simulink model "demo_interconnect_new"  (Simulink 7.4)
settings: Solver=ode45  StartTime=0.0  StopTime=100  RelTol=1e-3
undefined symbols (not defined in the file): ROACH
libraries: xbsIndex_r4 x58, isi_correlator_lib x22, xps_library x13, casper_library x8, dspsigops x8
settings Model: Creator=wjm  LastModifiedBy=wjm
settings OptimizationCC: InitFltsAndDblsToZero=on

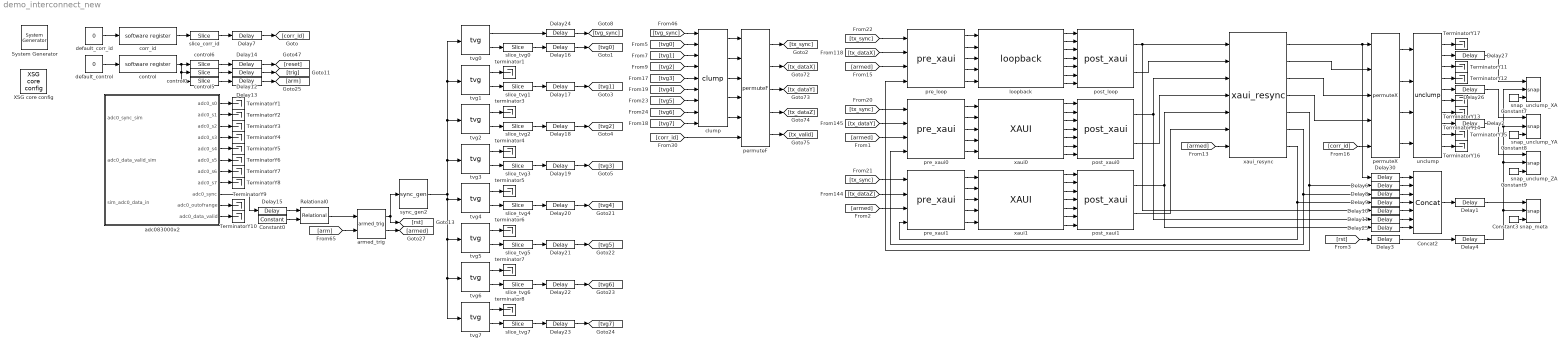
== system demo_interconnect_new ==
  " System Generator" : xbsIndex_r4/ System Generator  Tag=genX  SystemSampleTime=-1  xilinxfamily=virtex5  part=xc5vsx95t  speed=-1  package=ff1136  synthesis_tool=XST  clock_wrapper=Clock Enables  directory=./demo_interconnect_new/sysgen  testbench=off  simulink_period=1  sysclk_period=5  dcm_input_clock_period=100  incr_netlist=off  trim_vbits=Everywhere in SubSystem  dbl_ovrd=According to Block Masks  core_generation=According to Block Masks  run_coregen=off  deprecated_control=off  eval_field=0  block_type=sysgen
      settings: block_version=10.1.1
  Concat2 : xbsIndex_r4/Concat  num_inputs=7  dbl_ovrd=off  block_type=concat
      settings: block_version=11.3
  Constant0 : xbsIndex_r4/Constant  arith_type=Unsigned  const=0  n_bits=4  bin_pt=0  explicit_period=on  period=1  equ=P=C  opselect=C  inp2=PCIN>>17  opr=+  inp1=P  carry=CIN  dbl_ovrd=off  block_type=constant
  Constant{3,7..9} (4 alike) : xbsIndex_r4/Constant  arith_type=Boolean  const=1  n_bits=1  bin_pt=0  explicit_period=on  period=1  equ=P=C  opselect=C  inp2=PCIN>>17  opr=+  inp1=P  carry=CIN  dbl_ovrd=off  block_type=constant
      settings: block_version=10.1.1
  Delay{1..2,4,12..24,26..27} (18 alike) : xbsIndex_r4/Delay  en=off  latency=1  dbl_ovrd=off  reg_retiming=on  block_type=delay
  Delay{3,6,8..11,25,30} (8 alike) : xbsIndex_r4/Delay  en=off  latency=3  dbl_ovrd=off  reg_retiming=on  block_type=delay
  Delay7 : xbsIndex_r4/Delay  en=off  latency=0  dbl_ovrd=off  reg_retiming=on  block_type=delay
  Relational0 : xbsIndex_r4/Relational  mode=a!=b  en=off  latency=1  dbl_ovrd=off  block_type=relational
      settings: xl_area=[0, 0, 0, 0, 0, 0, 0]  block_version=10.1.3
  TerminatorY{1..17} (17 alike) : Terminator
  XSG core config : xps_library/XSG core config  Tag=xps:xsg  SystemSampleTime=-1  hw_sys=ROACH:sx95t  ibob_linux=off  clk_src=adc0_clk  iBOB_clk_src=sys_clk  BEE2_ctrl_clk_src=sys_clk  BEE2_usr_clk_src=sys_clk  ROACH_clk_src=adc0_clk  CORR_clk_src=sys_clk  gpio_clk_io_group=iBOB:sma  gpio_clk_bit_index=0  clk_rate=200  sample_period=1  synthesis_tool=XST  mpc_type=powerpc440_ext
  adc083000x2 : Subsystem  Tag=xps:adc083000x2  AncestorBlock=xps_library/adc083000x2  mask(adc_083000x2){use_adc0=on, use_adc1=off, demux_adc=off, clock_sync=off, verbose=off, using_ctrl=off, adc_clk_rate=800, sample_period=1, bit_width=8}
      mask prompts: use_adc0 "Use ZD0K0?"; use_adc1 "Use ZDOK1?"; demux_adc "Demux ADCs by 2?"; clock_sync "Interleave 2 ADC boards?"; verbose "Verbose Block Creation?"; using_ctrl "Add ports for control registers?"; adc_clk_rate "ADC clock rate (MHz)"; sample_period "Sample Period"; bit_width "Output Bit Width"
      mask help:
      | The ADC block converts analog inputs to digital outputs.
      | Every clock cycle, the inputs are sampled and digitized to
      | 8 bit binary point numbers in the range of [-1, 1).
      |
      | Online block-specific documentation: http://casper.berkeley.edu/wiki/Adc083000
      mask init:
      | adc083000_mask;
      mask Help: eval('xlWeb([getenv(''MLIB_ROOT''), ''\doc\html\sys_adc\sys_adc.html''])')
  armed_trig : isi_correlator_lib/armed_trig  SystemSampleTime=-1
  clump : isi_correlator_lib/clump  SystemSampleTime=-1
  control : xps_library/software register  Tag=xps:sw_reg  SystemSampleTime=-1  io_dir=From Processor  arith_type=Unsigned  bitwidth=32  bin_pt=0  sample_period=1  gw_name=demo_interconnect_new_control_user_data_out
  control0 : xbsIndex_r4/Slice  nbits=1  boolean_output=on  mode=Lower Bit Location + Width  bit1=0  base1=MSB of Input  bit0=0  base0=LSB of Input  dbl_ovrd=off  block_type=slice
      settings: infoedit="Extracts a given range of bits from each input sample and presents it at the output.  The output type is ordinarily unsigned with binary point at zero, but can be Boolean when the slice is one bit wide.<P><P>Hardware notes: In hardware this block costs nothing."  block_version=10.1.3
  control5 : xbsIndex_r4/Slice  nbits=1  boolean_output=on  mode=Lower Bit Location + Width  bit1=0  base1=MSB of Input  bit0=1  base0=LSB of Input  dbl_ovrd=off  block_type=slice
      settings: infoedit="Extracts a given range of bits from each input sample and presents it at the output.  The output type is ordinarily unsigned with binary point at zero, but can be Boolean when the slice is one bit wide.<P><P>Hardware notes: In hardware this block costs nothing."  block_version=10.1.3
  control6 : xbsIndex_r4/Slice  nbits=1  boolean_output=on  mode=Lower Bit Location + Width  bit1=0  base1=MSB of Input  bit0=2  base0=LSB of Input  dbl_ovrd=off  block_type=slice
      settings: infoedit="Extracts a given range of bits from each input sample and presents it at the output.  The output type is ordinarily unsigned with binary point at zero, but can be Boolean when the slice is one bit wide.<P><P>Hardware notes: In hardware this block costs nothing."  block_version=10.1.3
  corr_id : xps_library/software register  Tag=xps:sw_reg  SystemSampleTime=-1  io_dir=From Processor  arith_type=Unsigned  bitwidth=32  bin_pt=0  sample_period=1  gw_name=demo_interconnect_new_corr_id_user_data_out
  default_control : Constant  Value=0  OutDataType=sfix(16)  OutScaling=2^0  SampleTime=1
  default_corr_id : Constant  Value=0  OutDataType=sfix(16)  OutScaling=2^0  SampleTime=1
  loopback : isi_correlator_lib/loopback  SystemSampleTime=-1
  permuteF : isi_correlator_lib/permuteF  SystemSampleTime=-1  latency=3
  permuteX : isi_correlator_lib/permuteX  SystemSampleTime=-1  latency=3
  post_loop : isi_correlator_lib/post_xaui  SystemSampleTime=-1
  post_xaui0 : isi_correlator_lib/post_xaui  SystemSampleTime=-1
  post_xaui1 : isi_correlator_lib/post_xaui  SystemSampleTime=-1
  pre_loop : isi_correlator_lib/pre_xaui  SystemSampleTime=-1
  pre_xaui0 : isi_correlator_lib/pre_xaui  SystemSampleTime=-1
  pre_xaui1 : isi_correlator_lib/pre_xaui  SystemSampleTime=-1
  slice_corr_id : xbsIndex_r4/Slice  nbits=2  boolean_output=off  mode=Lower Bit Location + Width  bit1=0  base1=MSB of Input  bit0=0  base0=LSB of Input  dbl_ovrd=off  block_type=slice
      settings: infoedit="Extracts a given range of bits from each input sample and presents it at the output.  The output type is ordinarily unsigned with binary point at zero, but can be Boolean when the slice is one bit wide.<P><P>Hardware notes: In hardware this block costs nothing."  block_version=10.1.3
  slice_tvg{0..7} (8 alike) : xbsIndex_r4/Slice  nbits=8  boolean_output=off  mode=Lower Bit Location + Width  bit1=0  base1=MSB of Input  bit0=0  base0=LSB of Input  dbl_ovrd=off  block_type=slice
      settings: block_version=10.1.3
  snap_meta : casper_library/Scopes/snap  SystemSampleTime=-1  nsamples=13
  snap_unclump_XA : casper_library/Scopes/snap  SystemSampleTime=-1  nsamples=13
  snap_unclump_YA : casper_library/Scopes/snap  SystemSampleTime=-1  nsamples=13
  snap_unclump_ZA : casper_library/Scopes/snap  SystemSampleTime=-1  nsamples=13
  sync_gen2 : isi_correlator_lib/sync_gen  SystemSampleTime=-1
  terminator{1,3..8} (7 alike) : Terminator
  tvg{0..7} (8 alike) : isi_correlator_lib/tvg  SystemSampleTime=-1  length=2^11
  unclump : isi_correlator_lib/unclump  SystemSampleTime=-1
  xaui0 : xps_library/XAUI  Tag=xps:xaui  SystemSampleTime=-1  demux=2  port=ROACH:0  open_phy=off  show_param=off  pre_emph=3  swing=800
  xaui1 : xps_library/XAUI  Tag=xps:xaui  SystemSampleTime=-1  demux=2  port=ROACH:1  open_phy=off  show_param=off  pre_emph=3  swing=800
  xaui_resync : isi_correlator_lib/xaui_resync  SystemSampleTime=-1  depth=10
  wires:
  armed_trig/1 -> sync_gen2/1, [rst]
  armed_trig/2 -> [armed]
  [tvg_sync] -> clump/1
  [tvg0] -> clump/2
  [tvg1] -> clump/3
  [tvg2] -> clump/4
  [tvg3] -> clump/5
  [tvg4] -> clump/6
  [tvg5] -> clump/7
  [tvg6] -> clump/8
  tvg0/2 -> slice_tvg0/1
  tvg1/2 -> slice_tvg1/1
  tvg2/2 -> slice_tvg2/1
  tvg0/1 -> Delay24/1
  tvg1/1 -> terminator1/1
  tvg2/1 -> terminator3/1
  tvg7/2 -> slice_tvg7/1
  tvg5/2 -> slice_tvg5/1
  tvg6/2 -> slice_tvg6/1
  tvg4/2 -> slice_tvg4/1
  tvg3/2 -> slice_tvg3/1
  tvg3/1 -> terminator4/1
  tvg4/1 -> terminator5/1
  tvg5/1 -> terminator6/1
  tvg6/1 -> terminator7/1
  tvg7/1 -> terminator8/1
  slice_tvg0/1 -> Delay16/1
  slice_tvg1/1 -> Delay17/1
  slice_tvg2/1 -> Delay18/1
  slice_tvg3/1 -> Delay19/1
  slice_tvg4/1 -> Delay20/1
  slice_tvg5/1 -> Delay21/1
  slice_tvg6/1 -> Delay22/1
  slice_tvg7/1 -> Delay23/1
  permuteF/1 -> [tx_sync]
  permuteF/2 -> [tx_dataX]
  permuteF/3 -> [tx_dataY]
  permuteF/4 -> [tx_dataZ]
  permuteF/5 -> [tx_valid]
  [tvg7] -> clump/9
  clump/1 -> permuteF/1
  clump/2 -> permuteF/2
  clump/3 -> permuteF/3
  clump/4 -> permuteF/4
  clump/5 -> permuteF/5
  [corr_id] -> permuteF/6
  [arm] -> armed_trig/2
  default_corr_id/1 -> corr_id/1
  corr_id/1 -> slice_corr_id/1
  Delay7/1 -> [corr_id]
  slice_corr_id/1 -> Delay7/1
  default_control/1 -> control/1
  control6/1 -> Delay14/1
  control5/1 -> Delay12/1
  control0/1 -> Delay13/1
  control/1 -> control6/1, control0/1, control5/1
  Delay14/1 -> [reset]
  Delay12/1 -> [trig]
  Delay13/1 -> [arm]
  adc083000x2/1(adc0_s0) -> TerminatorY1/1
  adc083000x2/2(adc0_s1) -> TerminatorY2/1
  adc083000x2/3(adc0_s2) -> TerminatorY3/1
  adc083000x2/4(adc0_s3) -> TerminatorY4/1
  adc083000x2/5(adc0_s4) -> TerminatorY5/1
  adc083000x2/6(adc0_s5) -> TerminatorY6/1
  adc083000x2/7(adc0_s6) -> TerminatorY7/1
  adc083000x2/8(adc0_s7) -> TerminatorY8/1
  adc083000x2/10(adc0_outofrange) -> TerminatorY9/1
  adc083000x2/11(adc0_data_valid) -> TerminatorY10/1
  Constant0/1 -> Relational0/2
  adc083000x2/9(adc0_sync) -> Delay15/1
  Delay15/1 -> Relational0/1
  Relational0/1 -> armed_trig/1
  sync_gen2/1 -> tvg4/1, tvg5/1, tvg7/1, tvg6/1, tvg3/1, tvg2/1, tvg0/1, tvg1/1
  Delay16/1 -> [tvg0]
  Delay17/1 -> [tvg1]
  Delay18/1 -> [tvg2]
  Delay19/1 -> [tvg3]
  Delay20/1 -> [tvg4]
  Delay21/1 -> [tvg5]
  Delay22/1 -> [tvg6]
  Delay23/1 -> [tvg7]
  Delay24/1 -> [tvg_sync]
  Constant7/1 -> snap_unclump_XA/3
  Constant8/1 -> snap_unclump_YA/3
  Constant9/1 -> snap_unclump_ZA/3
  unclump/2 -> Delay27/1
  unclump/5 -> Delay26/1
  unclump/8 -> Delay2/1
  unclump/3 -> TerminatorY11/1
  unclump/4 -> TerminatorY12/1
  unclump/6 -> TerminatorY13/1
  unclump/7 -> TerminatorY14/1
  unclump/9 -> TerminatorY15/1
  unclump/10 -> TerminatorY16/1
  Delay2/1 -> snap_unclump_ZA/1
  Delay26/1 -> snap_unclump_YA/1
  Delay27/1 -> snap_unclump_XA/1
  Constant3/1 -> snap_meta/3
  Delay3/1 -> Delay4/1
  [rst] -> Delay3/1
  Concat2/1 -> Delay1/1
  Delay30/1 -> Concat2/1
  Delay6/1 -> Concat2/2
  Delay8/1 -> Concat2/3
  Delay9/1 -> Concat2/4
  Delay10/1 -> Concat2/5
  Delay11/1 -> Concat2/6
  Delay25/1 -> Concat2/7
  [corr_id] -> permuteX/5
  xaui_resync/1 -> permuteX/1, Delay30/1
  xaui_resync/2 -> permuteX/2
  xaui_resync/3 -> permuteX/3
  xaui_resync/4 -> permuteX/4
  [armed] -> xaui_resync/7
  xaui0/1 -> post_xaui0/1
  xaui0/2 -> post_xaui0/2
  xaui0/3 -> post_xaui0/3
  xaui0/4 -> post_xaui0/4
  xaui0/5 -> post_xaui0/5
  xaui0/6 -> post_xaui0/6
  xaui0/7 -> post_xaui0/7
  xaui1/1 -> post_xaui1/1
  xaui1/2 -> post_xaui1/2
  xaui1/3 -> post_xaui1/3
  xaui1/4 -> post_xaui1/4
  xaui1/5 -> post_xaui1/5
  xaui1/6 -> post_xaui1/6
  xaui1/7 -> post_xaui1/7
  [armed] -> pre_xaui0/3
  [tx_dataY] -> pre_xaui0/2
  [tx_sync] -> pre_xaui0/1
  [tx_sync] -> pre_xaui1/1
  [tx_dataZ] -> pre_xaui1/2
  pre_xaui0/1 -> xaui0/1
  pre_xaui0/2 -> xaui0/2
  pre_xaui0/3 -> xaui0/3
  pre_xaui0/4 -> xaui0/4
  pre_xaui0/5 -> xaui0/5
  pre_xaui1/1 -> xaui1/1
  pre_xaui1/2 -> xaui1/2
  pre_xaui1/3 -> xaui1/3
  pre_xaui1/4 -> xaui1/4
  pre_xaui1/5 -> xaui1/5
  [tx_dataX] -> pre_loop/2
  [armed] -> pre_loop/3
  [tx_sync] -> pre_loop/1
  xaui_resync/5 -> pre_loop/4, Delay6/1
  xaui_resync/6 -> pre_xaui0/4, Delay8/1
  xaui_resync/7 -> pre_xaui1/4, Delay9/1
  [armed] -> pre_xaui1/3
  pre_loop/1 -> loopback/1
  pre_loop/2 -> loopback/2
  pre_loop/3 -> loopback/3
  pre_loop/4 -> loopback/4
  pre_loop/5 -> loopback/5
  loopback/1 -> post_loop/1
  loopback/2 -> post_loop/2
  loopback/3 -> post_loop/3
  loopback/4 -> post_loop/4
  loopback/5 -> post_loop/5
  loopback/6 -> post_loop/6
  loopback/7 -> post_loop/7
  post_loop/2 -> xaui_resync/2
  post_xaui0/1 -> xaui_resync/3, Delay11/1
  post_xaui0/2 -> xaui_resync/4
  post_xaui1/1 -> xaui_resync/5, Delay25/1
  post_xaui1/2 -> xaui_resync/6
  post_loop/1 -> xaui_resync/1, Delay10/1
  permuteX/1 -> unclump/1
  permuteX/2 -> unclump/2
  permuteX/3 -> unclump/3
  permuteX/4 -> unclump/4
  unclump/1 -> TerminatorY17/1
  Delay1/1 -> snap_meta/1
  Delay4/1 -> snap_meta/2, snap_unclump_XA/2, snap_unclump_YA/2, snap_unclump_ZA/2

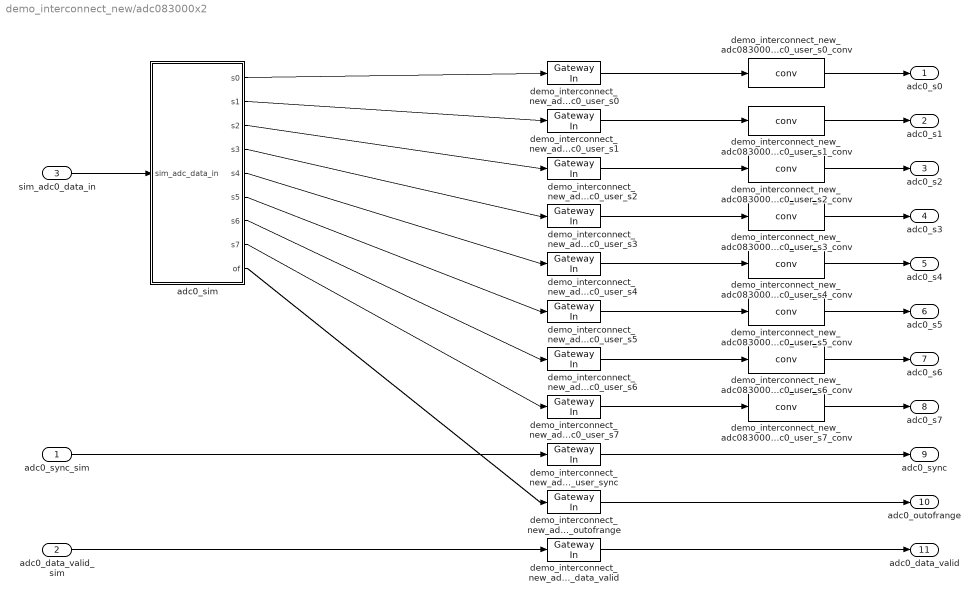
== system demo_interconnect_new/adc083000x2 ==
  adc0_sync_sim : Inport  OutDataType=sfix(16)  OutScaling=2^0
  adc0_data_valid_sim : Inport  Port=2  OutDataType=sfix(16)  OutScaling=2^0
  sim_adc0_data_in : Inport  Port=3  OutDataType=fixdt(1, 16)  OutScaling=2^0
  adc0_sim : Subsystem  AncestorBlock=xps_library/ADCs/adc_sim  mask(adc_sim){nStreams=8, bit_width=8}
      mask prompts: nStreams "Number of Output Streams"; bit_width "Sample Bit Width"
      mask help:
      | This block simulates the behavior of a demuxed ADC, which takes
      | as input a waveform and returns digital samples in parallel at
      | a slower rate.
      |
      | This block is used to simulate the behavior
      mask init:
      | adc_sim_init(gcb, ...
      |     'nStreams', nStreams, ...
      |     'bit_width', bit_width);
  demo_interconnect_new_adc083000x2_adc0_user_data_valid : xbsIndex_r4/Gateway In  arith_type=Unsigned  n_bits=1  bin_pt=0  quantization="Round  (unbiased: +/- Inf)"  overflow=Saturate  period=1  dbl_ovrd=off  timing_constraint=None  locs_specified=off  LOCs={}  hdl_port=on  block_type=gatewayin
      settings: infoedit="Gateway in block.  Converts inputs of type Simulink integer, double and fixed point to  Xilinx fixed point type.<br><br>Hardware notes:  In hardware these blocks become top level input ports."  block_version=11.4
  demo_interconnect_new_adc083000x2_adc0_user_outofrange : xbsIndex_r4/Gateway In  arith_type=Unsigned  n_bits=4  bin_pt=0  quantization="Round  (unbiased: +/- Inf)"  overflow=Saturate  period=1  dbl_ovrd=off  timing_constraint=None  locs_specified=off  LOCs={}  hdl_port=on  block_type=gatewayin
      settings: infoedit="Gateway in block.  Converts inputs of type Simulink integer, double and fixed point to  Xilinx fixed point type.<br><br>Hardware notes:  In hardware these blocks become top level input ports."  block_version=11.4
  demo_interconnect_new_adc083000x2_adc0_user_s{0..7} (8 alike) : xbsIndex_r4/Gateway In  arith_type=Unsigned  n_bits=8  bin_pt=0  quantization="Round  (unbiased: +/- Inf)"  overflow=Saturate  period=1  dbl_ovrd=off  timing_constraint=None  locs_specified=off  LOCs={}  hdl_port=on  block_type=gatewayin
      settings: infoedit="Gateway in block.  Converts inputs of type Simulink integer, double and fixed point to  Xilinx fixed point type.<br><br>Hardware notes:  In hardware these blocks become top level input ports."  block_version=11.4
  demo_interconnect_new_adc083000x2_adc0_user_s0_conv : xps_library/ADCs/conv  SystemSampleTime=-1  bit_width=8
  demo_interconnect_new_adc083000x2_adc0_user_s1_conv : xps_library/ADCs/conv  SystemSampleTime=-1  bit_width=8
  demo_interconnect_new_adc083000x2_adc0_user_s2_conv : xps_library/ADCs/conv  SystemSampleTime=-1  bit_width=8
  demo_interconnect_new_adc083000x2_adc0_user_s3_conv : xps_library/ADCs/conv  SystemSampleTime=-1  bit_width=8
  demo_interconnect_new_adc083000x2_adc0_user_s4_conv : xps_library/ADCs/conv  SystemSampleTime=-1  bit_width=8
  demo_interconnect_new_adc083000x2_adc0_user_s5_conv : xps_library/ADCs/conv  SystemSampleTime=-1  bit_width=8
  demo_interconnect_new_adc083000x2_adc0_user_s6_conv : xps_library/ADCs/conv  SystemSampleTime=-1  bit_width=8
  demo_interconnect_new_adc083000x2_adc0_user_s7_conv : xps_library/ADCs/conv  SystemSampleTime=-1  bit_width=8
  demo_interconnect_new_adc083000x2_adc0_user_sync : xbsIndex_r4/Gateway In  arith_type=Unsigned  n_bits=4  bin_pt=0  quantization="Round  (unbiased: +/- Inf)"  overflow=Saturate  period=1  dbl_ovrd=off  timing_constraint=None  locs_specified=off  LOCs={}  hdl_port=on  block_type=gatewayin
      settings: infoedit="Gateway in block.  Converts inputs of type Simulink integer, double and fixed point to  Xilinx fixed point type.<br><br>Hardware notes:  In hardware these blocks become top level input ports."  block_version=11.4
  adc0_s0 : Outport  OutDataType=fixdt(1, 16)  OutScaling=2^0
  adc0_s1 : Outport  Port=2  OutDataType=fixdt(1, 16)  OutScaling=2^0
  adc0_s2 : Outport  Port=3  OutDataType=fixdt(1, 16)  OutScaling=2^0
  adc0_s3 : Outport  Port=4  OutDataType=fixdt(1, 16)  OutScaling=2^0
  adc0_s4 : Outport  Port=5  OutDataType=fixdt(1, 16)  OutScaling=2^0
  adc0_s5 : Outport  Port=6  OutDataType=fixdt(1, 16)  OutScaling=2^0
  adc0_s6 : Outport  Port=7  OutDataType=fixdt(1, 16)  OutScaling=2^0
  adc0_s7 : Outport  Port=8  OutDataType=fixdt(1, 16)  OutScaling=2^0
  adc0_sync : Outport  Port=9  OutDataType=sfix(16)  OutScaling=2^0
  adc0_outofrange : Outport  Port=10  OutDataType=fixdt(1, 16)  OutScaling=2^0
  adc0_data_valid : Outport  Port=11  OutDataType=sfix(16)  OutScaling=2^0
  wires:
  sim_adc0_data_in/1 -> adc0_sim/1(sim_adc_data_in)
  adc0_sim/1(s0) -> demo_interconnect_new_adc083000x2_adc0_user_s0/1
  demo_interconnect_new_adc083000x2_adc0_user_s0/1 -> demo_interconnect_new_adc083000x2_adc0_user_s0_conv/1
  demo_interconnect_new_adc083000x2_adc0_user_s0_conv/1 -> adc0_s0/1
  adc0_sim/2(s1) -> demo_interconnect_new_adc083000x2_adc0_user_s1/1
  demo_interconnect_new_adc083000x2_adc0_user_s1/1 -> demo_interconnect_new_adc083000x2_adc0_user_s1_conv/1
  demo_interconnect_new_adc083000x2_adc0_user_s1_conv/1 -> adc0_s1/1
  adc0_sim/3(s2) -> demo_interconnect_new_adc083000x2_adc0_user_s2/1
  demo_interconnect_new_adc083000x2_adc0_user_s2/1 -> demo_interconnect_new_adc083000x2_adc0_user_s2_conv/1
  demo_interconnect_new_adc083000x2_adc0_user_s2_conv/1 -> adc0_s2/1
  adc0_sim/4(s3) -> demo_interconnect_new_adc083000x2_adc0_user_s3/1
  demo_interconnect_new_adc083000x2_adc0_user_s3/1 -> demo_interconnect_new_adc083000x2_adc0_user_s3_conv/1
  demo_interconnect_new_adc083000x2_adc0_user_s3_conv/1 -> adc0_s3/1
  adc0_sim/5(s4) -> demo_interconnect_new_adc083000x2_adc0_user_s4/1
  demo_interconnect_new_adc083000x2_adc0_user_s4/1 -> demo_interconnect_new_adc083000x2_adc0_user_s4_conv/1
  demo_interconnect_new_adc083000x2_adc0_user_s4_conv/1 -> adc0_s4/1
  adc0_sim/6(s5) -> demo_interconnect_new_adc083000x2_adc0_user_s5/1
  demo_interconnect_new_adc083000x2_adc0_user_s5/1 -> demo_interconnect_new_adc083000x2_adc0_user_s5_conv/1
  demo_interconnect_new_adc083000x2_adc0_user_s5_conv/1 -> adc0_s5/1
  adc0_sim/7(s6) -> demo_interconnect_new_adc083000x2_adc0_user_s6/1
  demo_interconnect_new_adc083000x2_adc0_user_s6/1 -> demo_interconnect_new_adc083000x2_adc0_user_s6_conv/1
  demo_interconnect_new_adc083000x2_adc0_user_s6_conv/1 -> adc0_s6/1
  adc0_sim/8(s7) -> demo_interconnect_new_adc083000x2_adc0_user_s7/1
  demo_interconnect_new_adc083000x2_adc0_user_s7/1 -> demo_interconnect_new_adc083000x2_adc0_user_s7_conv/1
  demo_interconnect_new_adc083000x2_adc0_user_s7_conv/1 -> adc0_s7/1
  adc0_sync_sim/1 -> demo_interconnect_new_adc083000x2_adc0_user_sync/1
  demo_interconnect_new_adc083000x2_adc0_user_sync/1 -> adc0_sync/1
  adc0_sim/9(of) -> demo_interconnect_new_adc083000x2_adc0_user_outofrange/1
  demo_interconnect_new_adc083000x2_adc0_user_outofrange/1 -> adc0_outofrange/1
  adc0_data_valid_sim/1 -> demo_interconnect_new_adc083000x2_adc0_user_data_valid/1
  demo_interconnect_new_adc083000x2_adc0_user_data_valid/1 -> adc0_data_valid/1

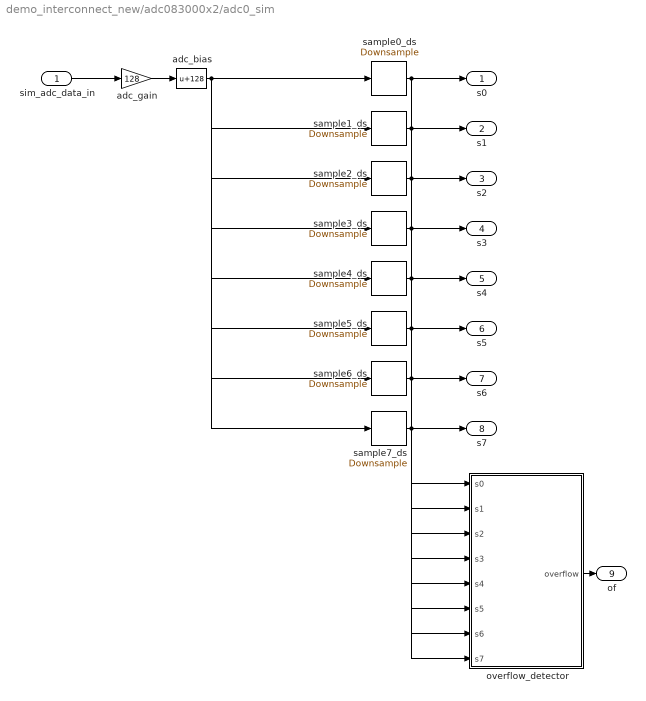
== system demo_interconnect_new/adc083000x2/adc0_sim ==
  sim_adc_data_in : Inport  OutDataType=sfix(16)  OutScaling=2^0
  adc_bias : Bias  Bias=128  SaturateOnIntegerOverflow=on
  adc_gain : Gain  Gain=128  ParameterDataType=sfix(16)  ParameterScaling=2^0  OutDataType=sfix(16)  OutScaling=2^0
  overflow_detector : Subsystem  AncestorBlock=casper_library/Misc/of_detect_bus  mask(of_detect_bus){nStreams=8, bit_width=8}
      mask prompts: nStreams "Number of Streams"; bit_width "Bit Width"
      mask init:
      | adc_overflow_detector_init(gcb, ...
      |     'nStreams', nStreams, ...
      |     'bit_width', bit_width);
  sample0_ds : dspsigops/Downsample  N=8  phase=1  ic=0  smode=Force single rate  fmode=Maintain input frame size
  sample1_ds : dspsigops/Downsample  N=8  phase=2  ic=0  smode=Force single rate  fmode=Maintain input frame size
  sample2_ds : dspsigops/Downsample  N=8  phase=3  ic=0  smode=Force single rate  fmode=Maintain input frame size
  sample3_ds : dspsigops/Downsample  N=8  phase=4  ic=0  smode=Force single rate  fmode=Maintain input frame size
  sample4_ds : dspsigops/Downsample  N=8  phase=5  ic=0  smode=Force single rate  fmode=Maintain input frame size
  sample5_ds : dspsigops/Downsample  N=8  phase=6  ic=0  smode=Force single rate  fmode=Maintain input frame size
  sample6_ds : dspsigops/Downsample  N=8  phase=7  ic=0  smode=Force single rate  fmode=Maintain input frame size
  sample7_ds : dspsigops/Downsample  N=8  phase=0  ic=0  smode=Force single rate  fmode=Maintain input frame size
  s0 : Outport  OutDataType=sfix(16)  OutScaling=2^0
  s1 : Outport  Port=2  OutDataType=sfix(16)  OutScaling=2^0
  s2 : Outport  Port=3  OutDataType=sfix(16)  OutScaling=2^0
  s3 : Outport  Port=4  OutDataType=sfix(16)  OutScaling=2^0
  s4 : Outport  Port=5  OutDataType=sfix(16)  OutScaling=2^0
  s5 : Outport  Port=6  OutDataType=sfix(16)  OutScaling=2^0
  s6 : Outport  Port=7  OutDataType=sfix(16)  OutScaling=2^0
  s7 : Outport  Port=8  OutDataType=sfix(16)  OutScaling=2^0
  of : Outport  Port=9  OutDataType=sfix(16)  OutScaling=2^0
  wires:
  sim_adc_data_in/1 -> adc_gain/1
  adc_gain/1 -> adc_bias/1
  overflow_detector/1(overflow) -> of/1
  adc_bias/1 -> sample0_ds/1, sample1_ds/1, sample2_ds/1, sample3_ds/1, sample4_ds/1, sample5_ds/1, sample6_ds/1, sample7_ds/1
  sample0_ds/1 -> overflow_detector/1(s0), s0/1
  sample1_ds/1 -> overflow_detector/2(s1), s1/1
  sample2_ds/1 -> overflow_detector/3(s2), s2/1
  sample3_ds/1 -> overflow_detector/4(s3), s3/1
  sample4_ds/1 -> overflow_detector/5(s4), s4/1
  sample5_ds/1 -> overflow_detector/6(s5), s5/1
  sample6_ds/1 -> overflow_detector/7(s6), s6/1
  sample7_ds/1 -> overflow_detector/8(s7), s7/1

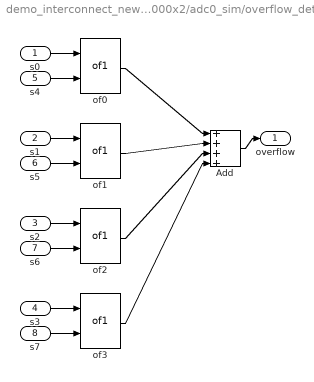
== system demo_interconnect_new/adc083000x2/adc0_sim/overflow_detector ==
  s0 : Inport  OutDataType=fixdt(1, 16)  OutScaling=2^0
  s1 : Inport  Port=2  OutDataType=fixdt(1, 16)  OutScaling=2^0
  s2 : Inport  Port=3  OutDataType=fixdt(1, 16)  OutScaling=2^0
  s3 : Inport  Port=4  OutDataType=fixdt(1, 16)  OutScaling=2^0
  s4 : Inport  Port=5  OutDataType=fixdt(1, 16)  OutScaling=2^0
  s5 : Inport  Port=6  OutDataType=fixdt(1, 16)  OutScaling=2^0
  s6 : Inport  Port=7  OutDataType=fixdt(1, 16)  OutScaling=2^0
  s7 : Inport  Port=8  OutDataType=fixdt(1, 16)  OutScaling=2^0
  Add : Sum  Inputs=++++  OutDataType=fixdt(1, 16)  OutScaling=2^-10
  of{0..3} (4 alike) : casper_library/Misc/of1  SystemSampleTime=-1  bit_num=0  n_adc_bits=8
  overflow : Outport  OutDataType=fixdt(1, 16)  OutScaling=2^0
  wires:
  s0/1 -> of0/1
  s4/1 -> of0/2
  of0/1 -> Add/1
  s1/1 -> of1/1
  s5/1 -> of1/2
  of1/1 -> Add/2
  s2/1 -> of2/1
  s6/1 -> of2/2
  of2/1 -> Add/3
  s3/1 -> of3/1
  s7/1 -> of3/2
  of3/1 -> Add/4
  Add/1 -> overflow/1
